simulink model "Approximierung"  (R2024a)
settings: Solver=VariableStepAuto  StartTime=0.0  StopTime=10.0  RelTol=1e-3
values from neighbouring files (symbols this model uses):
  K = K(:,:,VeloIndexK)    [loadSystem.m]
  relOutput = 1:1:length(K.InputName)    [loadSystem.m]
  sysCL = feedback(sysOL,K)    [loadSystem.m]
  sysOL = sysOL(relOutput,:,VeloIndexSys)    [loadSystem.m]
libraries: cstblocks x2
settings Model: Creator=sp-ma  LastModifiedBy=sp-ma

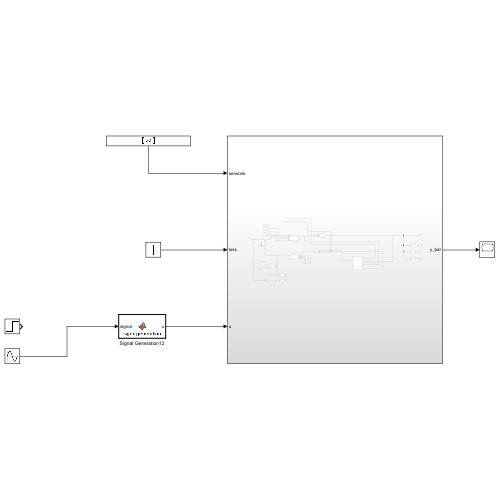
[thumbnail: Simulink's stored preview of the top-level diagram]
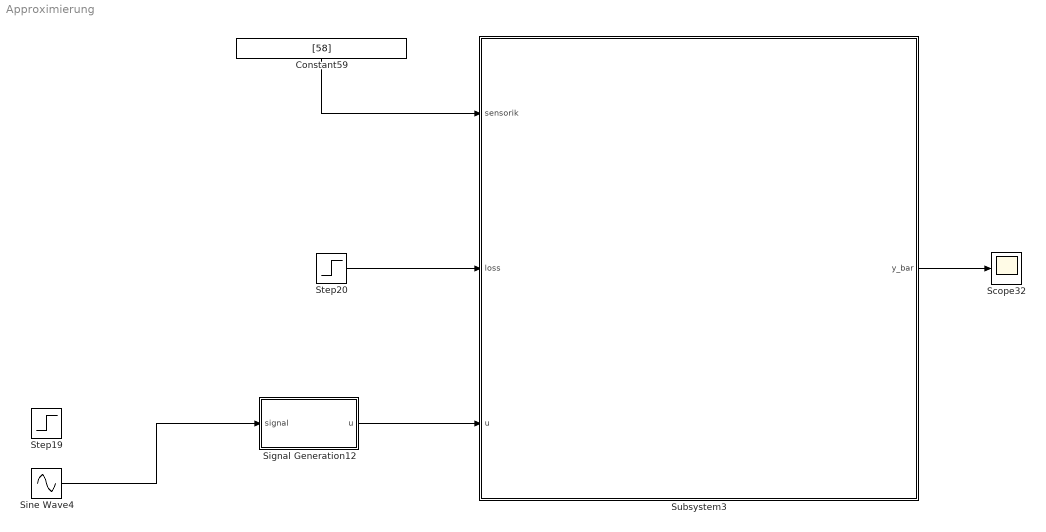
== system Approximierung ==
  Constant59 : Constant  Value=[58]
  Scope32 : Scope
  Signal Generation12 : MATLAB Function  TreatAsAtomicUnit=on
  Sine Wave4 : Sin  SampleTime=0
  Step19 : Step  Before=0.1  After=0.1  SampleTime=0
  Step20 : Step  Time=0.5  SampleTime=0
  Subsystem3 : Subsystem
  wires:
  Constant59/1 -> Subsystem3/1(sensorik)
  Step20/1 -> Subsystem3/2(loss)
  Signal Generation12/1(u) -> Subsystem3/3(u)
  Sine Wave4/1 -> Signal Generation12/1(signal)
  Subsystem3/1(y_bar) -> Scope32/1

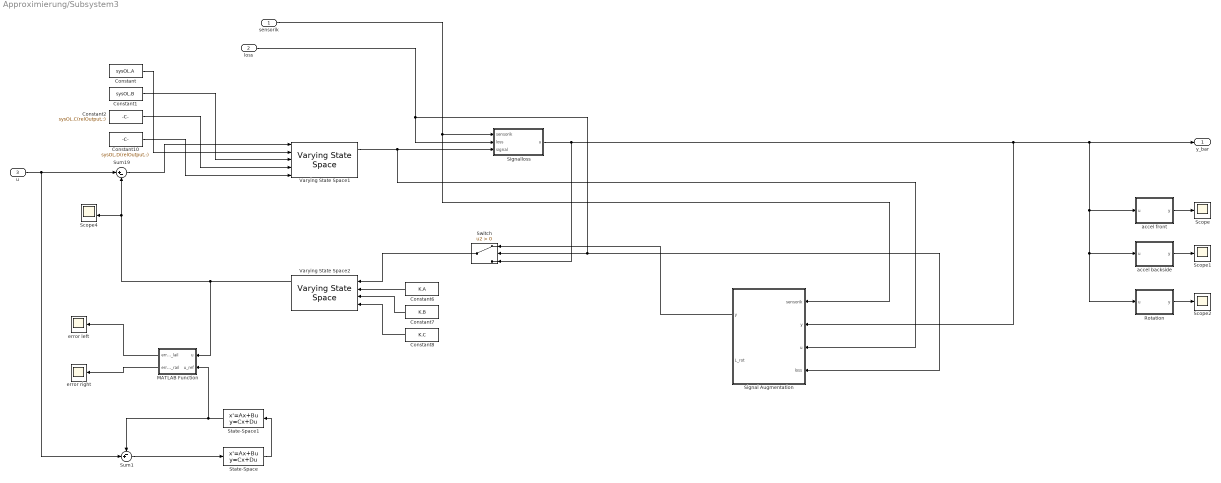
== system Approximierung/Subsystem3 ==
  sensorik : Inport
  loss : Inport  Port=2
  u : Inport  Port=3
  Constant : Constant  Value=sysOL.A  SampleTime=Inf
  Constant1 : Constant  Value=sysOL.B  SampleTime=Inf
  Constant10 : Constant  Value=sysOL.D(relOutput,:)
  Constant2 : Constant  Value=sysOL.C(relOutput,:)  SampleTime=Inf
  Constant6 : Constant  Value=K.A
  Constant7 : Constant  Value=K.B
  Constant8 : Constant  Value=K.C
  MATLAB Function : MATLAB Function  TreatAsAtomicUnit=on
  Rotation : MATLAB Function  TreatAsAtomicUnit=on
  Scope : Scope
  Scope1 : Scope
  Scope2 : Scope
  Scope4 : Scope  NumInputPorts=4
  Signal Augmentation : Subsystem
  Signalloss : MATLAB Function  TreatAsAtomicUnit=on
  State-Space : StateSpace  A=sysOL.A  B=sysOL.B  C=sysOL.C(relOutput,:)  D=sysCL.D(relOutput,:)  InitialCondition=0
  State-Space1 : StateSpace  A=K.A  B=K.B  C=K.C  D=K.D  InitialCondition=0
  Sum1 : Sum  Inputs=-+|
  Sum19 : Sum  Inputs=|+-
  Switch : Switch  Criteria=u2 > Threshold  SaturateOnIntegerOverflow=off  InputSameDT=off
  Varying State Space1 : cstblocks/Linear Parameter Varying/Varying State Space  x0=0  xNames=''  OutputX=on  OutputDX=on  Feedthrough=on  InputX0=off  InputDX0=off  InputU0=off  InputY0=off
  Varying State Space2 : cstblocks/Linear Parameter Varying/Varying State Space  x0=0  xNames=''  OutputX=on  OutputDX=on  Feedthrough=off  InputX0=off  InputDX0=off  InputU0=off  InputY0=off
  accel backside : MATLAB Function  TreatAsAtomicUnit=on
  accel front : MATLAB Function  TreatAsAtomicUnit=on
  error left : Scope
  error right : Scope
  y_bar : Outport
  wires:
  sensorik/1 -> Signalloss/1(sensorik), Signal Augmentation/1(sensorik)
  u/1 -> Sum1/2, Sum19/1
  Varying State Space1/1 -> Signalloss/3(signal), Signal Augmentation/3(u)
  Constant/1 -> Varying State Space1/2
  Constant1/1 -> Varying State Space1/3
  Constant2/1 -> Varying State Space1/4
  Constant10/1 -> Varying State Space1/5
  Sum19/1 -> Varying State Space1/1
  Varying State Space2/1 -> MATLAB Function/1(u), Sum19/2, Scope4/3
  Constant6/1 -> Varying State Space2/2
  Constant8/1 -> Varying State Space2/4
  Constant7/1 -> Varying State Space2/3
  Switch/1 -> Varying State Space2/1
  Rotation/1(y) -> Scope2/1
  accel backside/1(y) -> Scope1/1
  accel front/1(y) -> Scope/1
  Signalloss/1(u) -> Switch/3, accel front/1(u), accel backside/1(u), Rotation/1(u), y_bar/1, Signal Augmentation/2("y ")
  loss/1 -> Signal Augmentation/4(loss), Switch/2, Signalloss/2(loss)
  Signal Augmentation/1(y) -> Switch/1
  State-Space1/1 -> MATLAB Function/2(u_ref), Sum1/1
  Sum1/1 -> State-Space/1
  State-Space/1 -> State-Space1/1
  MATLAB Function/1(error_lail) -> error left/1
  MATLAB Function/2(error_rail) -> error right/1

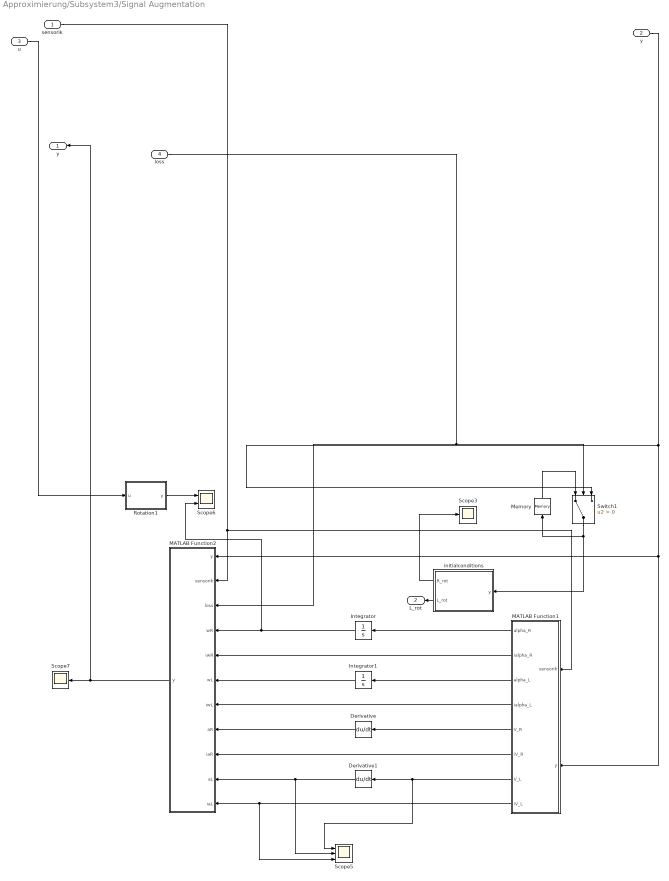
== system Approximierung/Subsystem3/Signal Augmentation ==
  sensorik : Inport
  "y " : Inport  Port=2
  u : Inport  Port=3
  loss : Inport  Port=4
  Derivative : Derivative
  Derivative1 : Derivative
  Integrator : Integrator
  Integrator1 : Integrator
  MATLAB Function1 : MATLAB Function  TreatAsAtomicUnit=on
  MATLAB Function2 : MATLAB Function  TreatAsAtomicUnit=on
  Memory : Memory
  Rotation1 : MATLAB Function  TreatAsAtomicUnit=on
  Scope3 : Scope
  Scope5 : Scope  NumInputPorts=3
  Scope6 : Scope  NumInputPorts=2
  Scope7 : Scope
  Switch1 : Switch  Criteria=u2 > Threshold  SaturateOnIntegerOverflow=off  InputSameDT=off
  initialconditions : Subsystem
  y : Outport
  L_rot : Outport  Port=2
  wires:
  MATLAB Function1/5(V_R) -> Derivative/1
  MATLAB Function1/6(iV_R) -> MATLAB Function2/9(iaR)
  MATLAB Function1/1(alpha_R) -> Integrator/1
  sensorik/1 -> MATLAB Function1/1(sensorik), MATLAB Function2/2(sensorik)
  u/1 -> Rotation1/1(u)
  MATLAB Function2/1(y) -> y/1, Scope7/1
  loss/1 -> Switch1/2, MATLAB Function2/3(loss)
  MATLAB Function1/2(ialpha_R) -> MATLAB Function2/5(iwR)
  initialconditions/2(R_rot) -> Scope3/1
  Switch1/1 -> Memory/1, initialconditions/1(y)
  MATLAB Function1/8(iV_L) -> Scope5/3, MATLAB Function2/11(iaL)
  Derivative1/1 -> Scope5/2, MATLAB Function2/10(aL)
  Integrator/1 -> Scope6/2, MATLAB Function2/4(wR)
  MATLAB Function1/4(ialpha_L) -> MATLAB Function2/7(iwL)
  MATLAB Function1/3(alpha_L) -> Integrator1/1
  MATLAB Function1/7(V_L) -> Scope5/1, Derivative1/1
  "y "/1 -> Switch1/3, MATLAB Function1/2(y), MATLAB Function2/1("y ")
  Memory/1 -> Switch1/1
  Derivative/1 -> MATLAB Function2/8(aR)
  Integrator1/1 -> MATLAB Function2/6(wL)
  Rotation1/1(y) -> Scope6/1
  initialconditions/1(L_rot) -> L_rot/1

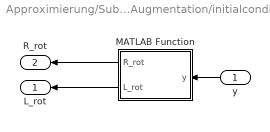
== system Approximierung/Subsystem3/Signal Augmentation/initialconditions ==
  y : Inport
  MATLAB Function : MATLAB Function  TreatAsAtomicUnit=on
  L_rot : Outport
  R_rot : Outport  Port=2
  wires:
  y/1 -> MATLAB Function/1(y)
  MATLAB Function/1(R_rot) -> R_rot/1
  MATLAB Function/2(L_rot) -> L_rot/1

== matlab function Approximierung/Subsystem3/Signal Augmentation/initialconditions/MATLAB Function ==
  data: y input; R_rot output; L_rot output
function [R_rot,L_rot] = fcn(y)
Lrot = [34 46 58];
Rrot = [70 82 94];
R_rot = y(Rrot)';
L_rot = y(Lrot)';

== matlab function Approximierung/Signal Generation12 ==
  data: u output; signal input
function u = signalgeneration(signal)
% t =0:10;
command = zeros(19,1);
% ilaileron = 13;
% iraileron = 14;
% command([15:19])=sin(t);
% % command([iraileron])=-1;

command([15 16]) = signal;
command([17 18]) = signal;
u=command;

== matlab function Approximierung/Subsystem3/Signal Augmentation/Rotation1 ==
  data: u input; y output
function y = fcn(u)
rot = [34 46 58 70 82 94];
y = u(rot);

== matlab function Approximierung/Subsystem3/Signalloss ==
  data: sensorik input; loss input; u output; signal input
function u = Signalloss(sensorik,loss,signal)

if(loss~=0)
    signal(sensorik)=0;
end
u=signal;

== matlab function Approximierung/Subsystem3/MATLAB Function ==
  data: u input; error_lail output; u_ref input; error_rail output
function [error_lail,error_rail] = fcn(u,u_ref)

error_lail = u(13)-u_ref(13);
error_rail = u(14)-u_ref(14);

== matlab function Approximierung/Subsystem3/accel front ==
  data: u input; y output
function y = fcn(u)
fw = [26 38 50 62 74 86];
y = u(fw);

== matlab function Approximierung/Subsystem3/accel backside ==
  data: u input; y output
function y = fcn(u)
bw = [32 44 56 68 80 92];
y = u(bw);

== matlab function Approximierung/Subsystem3/Rotation ==
  data: u input; y output
function y = fcn(u)
rot = [34 46 58 70 82 94];
y = u(rot);

== matlab function Approximierung/Subsystem3/Signal Augmentation/MATLAB Function1 ==
  data: sensorik input; alpha_R output; ialpha_R output; alpha_L output; ialpha_L output; y input; V_R output; iV_R output; V_L output; iV_L output
function [alpha_R,ialpha_R,alpha_L,ialpha_L,V_R,iV_R,V_L,iV_L] = fcn(sensorik,y)
    Rfw =  [62 74 86];
    Rbw =  [68 80 92];
    Rrot = [70 82 94];
    R = [Rfw;Rbw;Rrot];
    R_lookup=R;
    Lfw =  [26 38 50];
    Lbw =  [32 44 56];
    Lrot = [34 46 58];
    L = [Lfw;Lbw;Lrot];
    L_lookup=L;
    
    Rcoord=[415, 1061;...
            602, 1061;...
            789, 2121;...
            933, 2121;...
            1164, 3183;...
            1260, 3182];
    Lcoord=[415, -1061;...
            602, -1061;...
            789, -2123;...
            933, -2120;...
            1164, -3184;...
            1260, -3183];
    
    alpha_R=zeros(1,3);
    ialpha_R=zeros(1,3);
    alpha_L=zeros(1,3);
    ialpha_L=zeros(1,3);
    V_R=zeros(1,3);
    iV_R=zeros(1,3);
    V_L=zeros(1,3);
    iV_L=zeros(1,3);
    xR=[Rcoord(2,1)-Rcoord(1,1),Rcoord(4,1)-Rcoord(3,1),Rcoord(6,1)-Rcoord(5,1)]/10^3;
    xL=[Lcoord(2,1)-Lcoord(1,1),Lcoord(4,1)-Lcoord(3,1),Lcoord(6,1)-Lcoord(5,1)]/10^3;
    x=xR;
    
    %% Überprüfen ob mehr als ein Element in einer Sensorreihe fehlerhaft ist
    for l=1:length(sensorik)
        % indR = find(R==sensorik(l));
        R(R==sensorik(l))=0;
        % indL = find(L==sensorik(l));
        L(L==sensorik(l))=0;
    end
    % disp(R)
    % disp(L)
    
    %nachschauen welche Reihen ersetzt werden können
    numberR=3*ones(1,3);
    numberL=3*ones(1,3);
    for i=1:3
        numberR(i)=nnz(R(:,i));
        numberL(i)=nnz(L(:,i));
    end
    % disp(numberR)
    % disp(numberL)
    
    right=find(numberR==2);
    left=find(numberL==2);
    % disp(right)
    % disp(left)
    
    for l=1:length(right)
        row=find(R(:,right(l))==0);
        if row <=2
            V_R(l)=y(R(3,right(l)))*xR(right(l));
            iV_R(l)=R_lookup(row,right(l));
        elseif row==3
            alpha_R(l)=(y(R(2,right(l)))-y(R(1,right(l))))/xR(i);
            ialpha_R(l)=R_lookup(row,right(l));
        end
    end
    for l=1:length(left)
        row=find(L(:,left(l))==0);
        if find(L(:,left(l))==0)<=2
            V_L(l)=y(L(3,left(l)))*xL(left(l));
            iV_L(l)=L_lookup(row,left(l));
        elseif find(L(:,left(l))==0)==3
            alpha_L(l)=(y(L(2,left(l)))-y(L(1,left(l))))/xL(i);
            ialpha_L(l)=L_lookup(row,left(l));
        end
    end
end

== matlab function Approximierung/Subsystem3/Signal Augmentation/MATLAB Function2 ==
  data: y input; y output; sensorik input; loss input; wR input; iwR input; wL input; iwL input; aR input; iaR input; aL input; iaL input
function y = fcn(y, sensorik,loss,wR,iwR,wL,iwL,aR,iaR,aL,iaL)
Rfw =  [62 74 86];
Rbw =  [68 80 92];
Rrot = [70 82 94];
R=[Rfw;Rbw;Rrot];

Lfw =  [26 38 50];
Lbw =  [32 44 56];
Lrot = [34 46 58];
L=[Lfw;Lbw;Lrot];

if ~isempty(iaR)
    for l=1:length(iaR)
        [r,c]=find(R==iaR(l));
        if r==1
            y(R(r,c))=aR(l)+y(R(r+1,c));
        elseif r==2
            y(R(r,c))=y(R(r+1,c))-aR(l);
        end
    end
end
if ~isempty(iaL)
    for l=1:length(iaL)
        [r,c]=find(L==iaL(l));
        if r==1
            y(L(r,c))=aL(l)+y(L(r+1,c));
        elseif r==2
            y(L(r,c))=y(L(r+1,c))-aL(l);
        end
    end
end
if ~isempty(iwR)
    for l=1:length(iwR)
        [r,c]=find(R==iwR(l));
        y(R(r,c))=wR(l);
    end
end
if ~isempty(iwL)
    for l=1:length(iwL)
        [r,c]=find(L==iwL(l));
        y(L(r,c))=wL(l);
    end
end


% for l=1:length(sensorik)
%     if(sensorik(l)<60)
%         if ~isempty(find(Lfw==sensorik(l)))
%             index = Lfw==sensorik(l);
%             y(Lfw(index)) = aL(index)+y(Lbw(index));
%         elseif ~isempty(find(Lbw==sensorik(l)))
%             index = Lbw==sensorik(l);
%             y(Lbw(index)) = y(Lfw(index))-aL(index);
%         elseif ~isempty(find(Lrot==sensorik(l)))
%             index = Lrot==sensorik(l);
%             y(Lrot(index)) = VL(index);
%         end
%     elseif sensorik(l)>60
%         if ~isempty(find(Rfw==sensorik(l)))
%             index = Rfw==sensorik(l);
%             y(Rfw(index)) = aR(index)+y(Rbw(index));
%         elseif ~isempty(find(Rbw==sensorik(l)))
%             index = Rbw==sensorik(l);
%             y(Rbw(index)) = y(Rfw(index))-aR(index);
%         elseif ~isempty(find(Rrot==sensorik(l)))
%             index = Rrot==sensorik(l);
%             y(Rrot(index)) = VR(index);
%         end
%     end
% end
% 
% 
% 
y;
end
